simulink model "Vehicle_Model_WIP_V2"  (R2019b)
settings: Solver=FixedStepDiscrete  StartTime=0.0  StopTime=Simulink.t_end  FixedStep=Simulink.dt  RelTol=1e-3
undefined symbols (not defined in the file): BRK, BTRRAD, CHLR, CHRG, DCDC, DiscIntNeverNeededParam, FAN, INV, MTR, PTRAD, PUMP, Settings, TRSM, Vehicle, VHCL, WHL
libraries: simulink x9, EV_cooling x6, EV_VLD x5, EV_ePWT x5
(part 3 of 5)

== system Vehicle_Model_WIP_V2/VCU/Torque Request ==
  note: Regen Braking
  note: Coasting
  note: Regen Braking
  DRV_rThrottle : Inport
  DRV_rBrake : Inport  Port=2
  VLD_vActVhcl_kph : Inport  Port=3
  VCU_LimTrqFr_Nm : Inport  Port=4
  VCU_LimTrqRr_Nm : Inport  Port=5
  HMI_Cruise_kph : Inport  Port=6
  Abs : Abs
  Add : Sum
  BRK_Pct_Brk1 : Lookup_n-D  BreakpointsForDimension1=[0,0.1,0.2,0.5,0.75]  BreakpointsForDimension2=[0,18,72,135]  Table=reshape([0,0,0,0,0,0,0,0,0,0,1,0,0,0,0,1,0,0,0,0],5,4)  ExtrapMethod=Clip  UseLastTableValue=on  RndMeth=Simplest  InputSameDT=on
  Bias : Bias  Bias=-1
  Constant : Constant  Value=MTR.Front.Max_Torque_Nm
  Constant1 : Constant  Value=MTR.Rear.Max_Torque_Nm
  Gain1 : Gain  Gain=MTR.Front.Number_of_Motors
  Gain2 : Gain  Gain=MTR.Rear.Number_of_Motors
  Gain3 : Gain  Gain=MTR.Front.Number_of_Motors
  Gain4 : Gain  Gain=MTR.Rear.Number_of_Motors
  Product3 : Product  Inputs=3
  Product4 : Product  Inputs=3
  Regen : Subsystem  TreatAsAtomicUnit=on
  RegenCoeff : Constant  Value=0
  Saturation : Saturate  UpperLimit=VHCL.TrqDistr  LowerLimit=VHCL.TrqDistr
  Scope : Scope  NumInputPorts=2
  Sum : Sum  Inputs=+++
  Sum1 : Sum  Inputs=+++
  Terminator : Terminator
  TrqDstr : Subsystem  TreatAsAtomicUnit=on
  TrqDstrb MAP : Lookup_n-D  BreakpointsForDimension1=[0,350,500,2360]  BreakpointsForDimension2=[0,150,200,420]  Table=reshape([1,1,0.33,0.33,1,1,0.33,0.33,0.33,0.33,0.33,0.33,0.33,0.33,0.33,0.33],4,4)  InternalRulePriority=Speed  RndMeth=Simplest  InputSameDT=on
  TrqReqFr_Nm : Outport
  TrqReqRr_Nm : Outport  Port=2
  TrqDstrRr : Outport  Port=3
  VCU_rBrk : Outport  Port=4
  wires:
  DRV_rThrottle/1 -> [DRV_rThrottle]
  [DRV_rThrottle] -> TrqDstr/1(DRV_rThrottle)
  DRV_rBrake/1 -> [DRV_rBrake]
  VLD_vActVhcl_kph/1 -> [VLD_vAct]
  HMI_Cruise_kph/1 -> [HMI_Cruise]
  [HMI_Cruise] -> Terminator/1
  [DRV_rThrottle] -> BRK_Pct_Brk1/1
  [VLD_vAct] -> BRK_Pct_Brk1/2
  BRK_Pct_Brk1/1 -> Product3/2, Product4/2
  RegenCoeff/1 -> Product4/1, Product3/3
  [TrqReqFr] -> Sum/1
  [TrqReqRr] -> Sum1/2
  Constant/1 -> Gain3/1
  Constant1/1 -> Gain4/1
  [DRV_rBrake] -> Regen/1(DRV_rBrake)
  Regen/2(BrkTrqReqRr) -> [BrkTrqReqRr]
  Regen/1(BrkTrqReqFr) -> [BrkTrqReqFr]
  [BrkTrqReqFr] -> Sum/2
  Product4/1 -> Sum1/1
  Product3/1 -> Sum/3
  [BrkTrqReqRr] -> Sum1/3
  Regen/3(rBrk) -> VCU_rBrk/1
  [VLD_vAct] -> TrqDstrb MAP/2  "actual speed [km/h]"
  [VLD_vAct] -> Regen/2(VLD_vAct)
  TrqDstr/1(TrqReqFr) -> [TrqReqFr]
  TrqDstr/2(TrqReqRr) -> [TrqReqRr]
  Abs/1 -> TrqDstrRr/1
  Bias/1 -> Abs/1
  TrqDstrb MAP/1 -> Saturation/1  "Torque distribution FRONT [%]"
  [VCU_LimTrqFr_Nm] -> Gain1/1
  [VCU_LimTrqRr_Nm] -> Gain2/1
  [TrqDstrbFr] -> TrqDstr/2(TrqDistrFr)
  [TrqDstrbFr] -> Regen/3(TrqDistrFr)
  Add/1 -> TrqDstrb MAP/1  "Torque request [Nm]"
  Saturation/1 -> Bias/1, [TrqDstrbFr]
  VCU_LimTrqFr_Nm/1 -> [VCU_LimTrqFr_Nm]
  VCU_LimTrqRr_Nm/1 -> [VCU_LimTrqRr_Nm]
  Sum/1 -> Scope/1, TrqReqFr_Nm/1  "TrqReq_FrAxle_Nm"
  Sum1/1 -> Scope/2, TrqReqRr_Nm/1  "TrqReq_RrAxle_Nm"
  Gain1/1 -> Add/1  "Torque request [Nm]"
  Gain2/1 -> Add/2  "Torque request [Nm]"
  Gain3/1 -> Product3/1  "Torque request [Nm]"
  Gain4/1 -> Product4/3  "Torque request [Nm]"

== system Vehicle_Model_WIP_V2/VLD/Front Wheel Radius ==
  Vehicle Actual Speed [m/s] : Inport
  Weight Front [N] : Inport  Port=2
  " Wheel static radius under load" : Subsystem  Commented=on
  Constant{,1,10,15} (4 alike) : Constant
  Constant11 : Constant  Value=VHCL.Front.RollRadius_s1
  Constant12 : Constant  Value=VHCL.Front.RollRadius_s2
  Constant13 : Constant  Value=VHCL.Front.RollRadius_s3
  Constant14 : Constant  Value=VHCL.Front.RollRadius_s4
  Constant16 : Constant  Value=VHCL.Front.RollRadius_c
  Constant2 : Constant  Value=VHCL.Front.RollRadius_q1
  Constant3 : Constant  Value=VHCL.Front.RollRadius_p1
  Constant4 : Constant  Value=VHCL.Front.RollRadius_p2
  Constant5 : Constant  Value=VHCL.Front.RollRadius_p3
  Constant6 : Constant  Value=VHCL.Front.RollRadius_p4
  Constant7 : Constant  Value=VHCL.Front.RollRadius_q2
  Constant8 : Constant  Value=VHCL.Front.RollRadius_q3
  Constant9 : Constant  Value=VHCL.Front.RollRadius_q4
  Divide{1..19} (19 alike) : Product
  Gain : Gain  Gain=0.5
  Goto2 : Goto  Commented=on  GotoTag=LVD_RFrStc_m
  Subtract : Sum  Inputs=4
  Subtract1 : Sum  Inputs=4
  Subtract2 : Sum  Inputs=4
  Subtract3 : Sum  Inputs=3
  LVD_RWhlFr_m : Outport  VectorParamsAs1DForOutWhenUnconnected=off
  wires:
  [LVD_RWhlFr_m] -> LVD_RWhlFr_m/1
  Vehicle Actual Speed [m/s]/1 -> [v_mps]
  " Wheel static radius under load"/1(LVD_RFrStc_m) -> Goto2/1
  Subtract3/1 -> Divide19/2
  [v_mps] -> Divide2/1, Divide2/2
  Divide2/1 -> [v_mps_2]
  Divide4/1 -> [W_N_3]
  Divide5/1 -> Divide4/1, [W_N_2]
  [W_N] -> Divide5/2, Divide4/2, Divide5/1
  Constant3/1 -> Divide1/1
  [W_N_3] -> Divide1/2
  [W_N_2] -> Divide6/2
  Constant4/1 -> Divide6/1
  Constant6/1 -> Divide8/1
  Constant/1 -> Divide8/2
  [W_N] -> Divide7/2
  Constant5/1 -> Divide7/1
  Divide1/1 -> Subtract/1
  Divide6/1 -> Subtract/2
  Divide7/1 -> Subtract/3
  Divide8/1 -> Subtract/4
  Subtract/1 -> Divide9/1
  [v_mps_2] -> Divide9/2
  [v_mps] -> Divide13/2
  Subtract1/1 -> Divide13/1
  Divide12/1 -> Subtract1/4
  Divide11/1 -> Subtract1/3
  Divide10/1 -> Subtract1/2
  Divide3/1 -> Subtract1/1
  Constant8/1 -> Divide11/1
  [W_N] -> Divide11/2
  Constant1/1 -> Divide12/2
  Constant9/1 -> Divide12/1
  Constant7/1 -> Divide10/1
  [W_N_2] -> Divide10/2
  [W_N_3] -> Divide3/2
  Constant2/1 -> Divide3/1
  Constant11/1 -> Divide18/1
  [W_N_3] -> Divide18/2
  [W_N_2] -> Divide14/2
  Constant12/1 -> Divide14/1
  Constant14/1 -> Divide16/1
  Constant10/1 -> Divide16/2
  [W_N] -> Divide15/2
  Constant13/1 -> Divide15/1
  Divide18/1 -> Subtract2/1
  Divide14/1 -> Subtract2/2
  Divide15/1 -> Subtract2/3
  Divide16/1 -> Subtract2/4
  Subtract2/1 -> Divide17/1
  Constant15/1 -> Divide17/2
  Divide9/1 -> Subtract3/1
  Divide13/1 -> Subtract3/2
  Divide17/1 -> Subtract3/3
  Divide19/1 -> [LVD_RWhlFr_m]
  Constant16/1 -> Divide19/1
  Weight Front [N]/1 -> Gain/1
  Gain/1 -> [W_N]

== system Vehicle_Model_WIP_V2/VLD/Inertia ==
  note: Rear
  note: Front
  TRSM_tauFrt : Inport
  TRSM_tauRr : Inport  Port=2
  Add5 : Sum  Inputs=3
  Add6 : Sum  Inputs=3
  Constant1 : Constant  Value=MTR.Front.Number_of_Motors
  Constant11 : Constant  Value=TRSM.Front.Inertia_kgm2
  Constant12 : Constant  Value=TRSM.Rear.Inertia_kgm2
  Constant13 : Constant  Value=MTR.Rear.Inertia_kgm2
  Constant14 : Constant  Value=WHL.Rear.Inertia_kgm2
  Constant2 : Constant  Value=MTR.Rear.Number_of_Motors
  Constant3 : Constant  Value=MTR.Front.Number_of_Motors
  Constant4 : Constant  Value=MTR.Rear.Number_of_Motors
  Constant8 : Constant  Value=MTR.Front.Inertia_kgm2
  Constant9 : Constant  Value=WHL.Front.Inertia_kgm2
  Divide{1,5,8,10} (4 alike) : Product
  Divide{2..3,7,11} (4 alike) : Product  Inputs=3
  Gain2 : Gain  Gain=2
  Gain3 : Gain  Gain=2
  VLD_FrtInrt_kgm2 : Outport  VectorParamsAs1DForOutWhenUnconnected=off
  VLD_RrInrt_kgm2 : Outport  Port=2  VectorParamsAs1DForOutWhenUnconnected=off
  wires:
  TRSM_tauFrt/1 -> [TRSM_tauFrt]
  TRSM_tauRr/1 -> [TRSM_tauRr]
  Divide5/1 -> Divide7/1
  Constant8/1 -> Divide7/2
  [TRSM_tauFrt] -> Divide5/2, Divide5/1
  Divide1/1 -> Divide2/1
  [TRSM_tauFrt] -> Divide1/1, Divide1/2
  Constant11/1 -> Divide2/2
  Constant9/1 -> Gain2/1
  Divide2/1 -> Add5/2
  Gain2/1 -> Add5/3
  Divide7/1 -> Add5/1
  Constant14/1 -> Gain3/1
  Divide11/1 -> Add6/1
  Constant13/1 -> Divide11/2
  [TRSM_tauRr] -> Divide8/1, Divide8/2
  Gain3/1 -> Add6/3
  Divide10/1 -> Divide11/1
  [TRSM_tauRr] -> Divide10/2, Divide10/1
  Add5/1 -> [VLD_FrtInrt_kgm2]
  Add6/1 -> [VLD_RrInrt_kgm2]
  [VLD_RrInrt_kgm2] -> VLD_RrInrt_kgm2/1
  [VLD_FrtInrt_kgm2] -> VLD_FrtInrt_kgm2/1
  Constant1/1 -> Divide7/3
  Constant2/1 -> Divide11/3
  Constant3/1 -> Divide2/3
  Divide3/1 -> Add6/2
  Constant12/1 -> Divide3/2
  Divide8/1 -> Divide3/1
  Constant4/1 -> Divide3/3

== system Vehicle_Model_WIP_V2/VLD/Rear Wheel Radius ==
  Vehicle Actual Speed [m/s] : Inport
  Weight Rear [N] : Inport  Port=2
  " Wheel static radius under load" : Subsystem  Commented=on
  Constant{,1,10,15} (4 alike) : Constant
  Constant11 : Constant  Value=VHCL.Rear.RollRadius_s1
  Constant12 : Constant  Value=VHCL.Rear.RollRadius_s2
  Constant13 : Constant  Value=VHCL.Rear.RollRadius_s3
  Constant14 : Constant  Value=VHCL.Rear.RollRadius_s4
  Constant16 : Constant  Value=VHCL.Rear.RollRadius_c
  Constant2 : Constant  Value=VHCL.Rear.RollRadius_q1
  Constant3 : Constant  Value=VHCL.Rear.RollRadius_p1
  Constant4 : Constant  Value=VHCL.Rear.RollRadius_p2
  Constant5 : Constant  Value=VHCL.Rear.RollRadius_p3
  Constant6 : Constant  Value=VHCL.Rear.RollRadius_p4
  Constant7 : Constant  Value=VHCL.Rear.RollRadius_q2
  Constant8 : Constant  Value=VHCL.Rear.RollRadius_q3
  Constant9 : Constant  Value=VHCL.Rear.RollRadius_q4
  Divide{1..19} (19 alike) : Product
  Gain : Gain  Gain=0.5
  Goto2 : Goto  Commented=on  GotoTag=LVD_RFrStc_m
  Subtract : Sum  Inputs=4
  Subtract1 : Sum  Inputs=4
  Subtract2 : Sum  Inputs=4
  Subtract3 : Sum  Inputs=3
  LVD_RWhlRr_m : Outport  VectorParamsAs1DForOutWhenUnconnected=off
  wires:
  [LVD_RWhlFr_m] -> LVD_RWhlRr_m/1
  Vehicle Actual Speed [m/s]/1 -> [v_mps]
  " Wheel static radius under load"/1(LVD_RFrStc_m) -> Goto2/1
  [v_mps] -> Divide2/1, Divide2/2
  Divide2/1 -> [v_mps_2]
  Divide4/1 -> [W_N_3]
  Divide5/1 -> Divide4/1, [W_N_2]
  [W_N] -> Divide5/2, Divide4/2, Divide5/1
  Constant3/1 -> Divide1/1
  [W_N_3] -> Divide1/2
  [W_N_2] -> Divide6/2
  Constant4/1 -> Divide6/1
  Constant6/1 -> Divide8/1
  Constant/1 -> Divide8/2
  [W_N] -> Divide7/2
  Constant5/1 -> Divide7/1
  Divide1/1 -> Subtract/1
  Divide6/1 -> Subtract/2
  Divide7/1 -> Subtract/3
  Divide8/1 -> Subtract/4
  Subtract/1 -> Divide9/1
  [v_mps_2] -> Divide9/2
  [v_mps] -> Divide13/2
  Subtract1/1 -> Divide13/1
  Divide12/1 -> Subtract1/4
  Divide11/1 -> Subtract1/3
  Divide10/1 -> Subtract1/2
  Divide3/1 -> Subtract1/1
  Constant8/1 -> Divide11/1
  [W_N] -> Divide11/2
  Constant1/1 -> Divide12/2
  Constant9/1 -> Divide12/1
  Constant7/1 -> Divide10/1
  [W_N_2] -> Divide10/2
  [W_N_3] -> Divide3/2
  Constant2/1 -> Divide3/1
  Constant11/1 -> Divide18/1
  [W_N_3] -> Divide18/2
  [W_N_2] -> Divide14/2
  Constant12/1 -> Divide14/1
  Constant14/1 -> Divide16/1
  Constant10/1 -> Divide16/2
  [W_N] -> Divide15/2
  Constant13/1 -> Divide15/1
  Divide18/1 -> Subtract2/1
  Divide14/1 -> Subtract2/2
  Divide15/1 -> Subtract2/3
  Divide16/1 -> Subtract2/4
  Subtract2/1 -> Divide17/1
  Constant15/1 -> Divide17/2
  Divide9/1 -> Subtract3/1
  Divide13/1 -> Subtract3/2
  Divide17/1 -> Subtract3/3
  Divide19/1 -> [LVD_RWhlFr_m]
  Constant16/1 -> Divide19/1
  Subtract3/1 -> Divide19/2
  Weight Rear [N]/1 -> Gain/1
  Gain/1 -> [W_N]

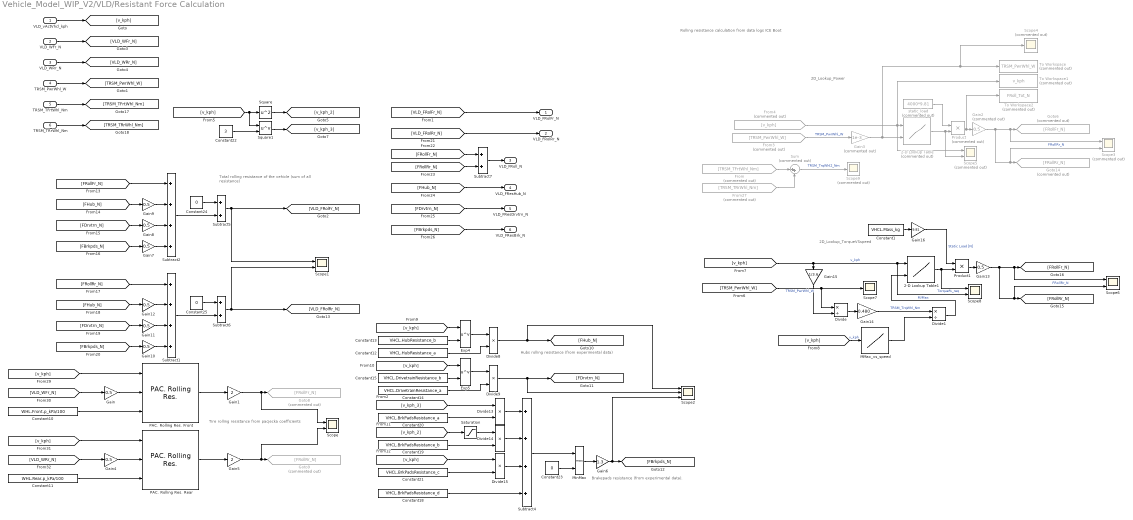
== system Vehicle_Model_WIP_V2/VLD/Resistant Force Calculation ==
  note: Rolling resistance calculation from data logs ICE Boot
  note: 2D_Lookup_Power
  note: Hubs rolling resistance (from experimental data)
  note: Brakepads resistance (from experimental data).
  note: Tire rolling resistance from pacjecka coefficients
  note: Total rolling resistance of the vehicle (sum of all resistance)
  note: 2D_Lookup_TorqueVSspeed
  VLD_vActVhcl_kph : Inport
  VLD_WFr_N : Inport  Port=2
  VLD_WRr_N : Inport  Port=3
  TRSM_PwrWhl_W : Inport  Port=4
  TRSM_TFrtWhl_Nm : Inport  Port=5
  TRSM_TRrWhl_Nm : Inport  Port=6
  2-D Lookup Table : Lookup_n-D  Commented=on  BreakpointsForDimension1=[0,1,18,54,72,162]  BreakpointsForDimension2=[0,250]  Table=reshape([0,0.23,0.23,0.18,0.15,0.15,0.68,0.68,0.68,0.3,0.3,0.3],6,2)  ExtrapMethod=Clip  InternalRulePriority=Speed  RndMeth=Simplest  InputSameDT=on
  2-D Lookup Table1 : Lookup_n-D  BreakpointsForDimension1=[0,1,18,54,72,162]  BreakpointsForDimension2=[0,1.4,2]  Table=reshape([0,0.23,0.23,0.18,0.15,0.15,0.68,0.68,0.68,0.3,0.3,0.3,0.75,0.75,0.75,0.35,0.35,0.35],6,3)  ExtrapMethod=Clip  InternalRulePriority=Speed  RndMeth=Simplest  InputSameDT=on
  Constant1 : Constant  Value=VHCL.Mass_kg  VectorParams1D=off
  Constant10 : Constant  Value=WHL.Front.p_kPa/100
  Constant11 : Constant  Value=WHL.Rear.p_kPa/100
  Constant12 : Constant  Value=VHCL.HubResistance_a
  Constant13 : Constant  Value=VHCL.HubResistance_b
  Constant14 : Constant  Value=VHCL.DrivetrainResistance_a
  Constant15 : Constant  Value=VHCL.DrivetrainResistance_b
  Constant18 : Constant  Value=VHCL.BrkPadsResistance_d
  Constant19 : Constant  Value=VHCL.BrkPadsResistance_b
  Constant20 : Constant  Value=VHCL.BrkPadsResistance_a
  Constant21 : Constant  Value=VHCL.BrkPadsResistance_c
  Constant22 : Constant  Value=3
  Constant23 : Constant  Value=0
  Constant24 : Constant  Value=0
  Constant25 : Constant  Value=0
  Divide : Product  Inputs=*/
  Divide1 : Product  Inputs=*/
  Divide{8..9,13..15} (5 alike) : Product
  Exp4 : Math  Operator=pow  SignedPower=off  SaturateOnIntegerOverflow=on
  Exp5 : Math  Operator=pow  SignedPower=off  SaturateOnIntegerOverflow=on
  From : From  Commented=on  GotoTag=TRSM_TFrtWhl_Nm
  From27 : From  Commented=on  GotoTag=TRSM_TRrWhl_Nm
  From3 : From  Commented=on  GotoTag=TRSM_PwrWhl_W
  From4 : From  Commented=on  GotoTag=v_kph
  Gain{,4,7..13} (9 alike) : Gain  Gain=0.5
  Gain1 : Gain  Gain=2
  Gain14 : Gain  Gain=0.480
  Gain15 : Gain  Gain=1/3.6
  Gain16 : Gain  Gain=9.81
  Gain2 : Gain  Commented=on  Gain=0.5
  Gain3 : Gain  Commented=on  Gain=1e-3
  Gain5 : Gain  Gain=2
  Gain6 : Gain  Gain=1.3
  Goto14 : Goto  Commented=on  GotoTag=FRollRr_N
  Goto6 : Goto  Commented=on  GotoTag=FRollFr_N
  Goto8 : Goto  Commented=on  GotoTag=FRollFr_N
  Goto9 : Goto  Commented=on  GotoTag=FRollRr_N
  MMax_vs_speed : Lookup_n-D  NumberOfTableDimensions=1  BreakpointsForDimension1=[0 5 10 15 20 25 30 35 40 45]*3.6  Table=[17000 17000 9500 7500 5750 4750 4000 3250 2800 2500]  ExtrapMethod=Clip  InternalRulePriority=Speed  RndMeth=Simplest  InputSameDT=on
  MinMax : MinMax  Function=max  Inputs=2
  PAC. Rolling Res. Front : EV_VLD/PAC. Rolling Res.  Vref_kmph=VHCL.RollResistance_V0  Fzref_N=VHCL.RollResistance_Fz0  pref_bar=VHCL.RollResistance_p0  SF=VHCL.Front.CRRgain  qsy1=VHCL.RollResistance_qsy1  qsy2=VHCL.RollResistance_qsy2  qsy3=VHCL.RollResistance_qsy3  qsy4=VHCL.RollResistance_qsy4  qsy5=VHCL.RollResistance_qsy5  qsy6=VHCL.RollResistance_qsy6  qsy7=VHCL.RollResistance_qsy7  qsy8=VHCL.RollResistance_qsy8
      settings: SourceProductName=EV_lib
  PAC. Rolling Res. Rear : EV_VLD/PAC. Rolling Res.  Vref_kmph=VHCL.RollResistance_V0  Fzref_N=VHCL.RollResistance_Fz0  pref_bar=VHCL.RollResistance_p0  SF=VHCL.Rear.CRRgain  qsy1=VHCL.RollResistance_qsy1  qsy2=VHCL.RollResistance_qsy2  qsy3=VHCL.RollResistance_qsy3  qsy4=VHCL.RollResistance_qsy4  qsy5=VHCL.RollResistance_qsy5  qsy6=VHCL.RollResistance_qsy6  qsy7=VHCL.RollResistance_qsy7  qsy8=VHCL.RollResistance_qsy8
      settings: SourceProductName=EV_lib
  Product : Product  Commented=on
  Product1 : Product
  Saturation : Saturate  UpperLimit=150*150  LowerLimit=0
  Scope{,1,6,8} (4 alike) : Scope  NumInputPorts=2
  Scope2 : Scope  NumInputPorts=3
  Scope3 : Scope  Commented=on  NumInputPorts=2
  Scope4 : Scope  Commented=on
  Scope5 : Scope  Commented=on  NumInputPorts=2
  Scope7 : Scope
  Scope9 : Scope  Commented=on
  Square : Math  Operator=square  SignedPower=off  SaturateOnIntegerOverflow=on
  Square1 : Math  Operator=pow  SignedPower=off  SaturateOnIntegerOverflow=on
  Subtract1 : Sum  Inputs=++++
  Subtract2 : Sum  Inputs=++++
  Subtract4 : Sum  Inputs=++++
  Subtract5 : Sum
  Subtract6 : Sum
  Subtract7 : Sum
  Sum : Sum  Commented=on  Inputs=|++
  To Workspace : ToWorkspace  Commented=on  VariableName=TRSM_PwrWhl_W  SaveFormat=Timeseries  SampleTime=-1
  To Workspace1 : ToWorkspace  Commented=on  VariableName=v_kph  SaveFormat=Timeseries  SampleTime=-1
  To Workspace2 : ToWorkspace  Commented=on  VariableName=FRoll_Tot_N  SaveFormat=Timeseries  SampleTime=-1
  static_load : Constant  Commented=on  Value=4000*9.81
  VLD_FRolFr_N : Outport  VectorParamsAs1DForOutWhenUnconnected=off
  VLD_FRolRr_N : Outport  Port=2  VectorParamsAs1DForOutWhenUnconnected=off
  VLD_FRoll_N : Outport  Port=3  VectorParamsAs1DForOutWhenUnconnected=off
  VLD_FResHub_N : Outport  Port=4  VectorParamsAs1DForOutWhenUnconnected=off
  VLD_FResDrvtrn_N : Outport  Port=5  VectorParamsAs1DForOutWhenUnconnected=off
  VLD_FResBrk_N : Outport  Port=6  VectorParamsAs1DForOutWhenUnconnected=off
  wires:
  VLD_vActVhcl_kph/1 -> [v_kph]
  [VLD_FRolFr_N] -> VLD_FRolFr_N/1
  [v_kph] -> Square1/1, Square/1
  Square/1 -> [v_kph_2]
  VLD_WFr_N/1 -> [VLD_WFr_N]
  VLD_WRr_N/1 -> [VLD_WRr_N]
  Constant12/1 -> Divide8/2
  [v_kph] -> Exp4/1
  Constant13/1 -> Exp4/2
  Exp4/1 -> Divide8/1
  Exp5/1 -> Divide9/1
  Constant15/1 -> Exp5/2
  [v_kph] -> Exp5/1
  Constant14/1 -> Divide9/2
  Constant18/1 -> Subtract4/4
  Divide13/1 -> Subtract4/1
  Divide14/1 -> Subtract4/2
  [v_kph_2] -> Saturation/1
  Constant19/1 -> Divide14/2
  Constant20/1 -> Divide13/2
  [v_kph_3] -> Divide13/1
  Constant21/1 -> Divide15/2
  [v_kph] -> Divide15/1
  Divide15/1 -> Subtract4/3
  Square1/1 -> [v_kph_3]
  Constant22/1 -> Square1/2
  MinMax/1 -> Gain6/1
  Subtract4/1 -> MinMax/1
  Constant23/1 -> MinMax/2
  Subtract5/1 -> [VLD_FRolFr_N], Scope1/1
  Subtract2/1 -> Subtract5/2
  Constant24/1 -> Subtract5/1
  Divide8/1 -> [FHub_N], Scope2/1
  Divide9/1 -> [FDrvtrn_N], Scope2/2
  Gain6/1 -> [FBrkpds_N], Scope2/3
  [FRollFr_N] -> Subtract2/1
  [FHub_N] -> Gain9/1
  [FDrvtrn_N] -> Gain8/1
  [FBrkpds_N] -> Gain7/1
  Gain7/1 -> Subtract2/4
  Gain8/1 -> Subtract2/3
  Gain9/1 -> Subtract2/2
  Gain12/1 -> Subtract1/2
  Gain11/1 -> Subtract1/3
  Gain10/1 -> Subtract1/4
  [FBrkpds_N] -> Gain10/1
  [FDrvtrn_N] -> Gain11/1
  [FHub_N] -> Gain12/1
  [FRollRr_N] -> Subtract1/1
  Constant25/1 -> Subtract6/1
  Subtract1/1 -> Subtract6/2
  Subtract6/1 -> [VLD_FRolRr_N], Scope1/2
  [VLD_FRolRr_N] -> VLD_FRolRr_N/1
  [FRollRr_N] -> Subtract7/2
  [FRollFr_N] -> Subtract7/1
  Subtract7/1 -> VLD_FRoll_N/1
  Saturation/1 -> Divide14/1
  [FHub_N] -> VLD_FResHub_N/1
  [FDrvtrn_N] -> VLD_FResDrvtrn_N/1
  [FBrkpds_N] -> VLD_FResBrk_N/1
  [v_kph] -> PAC. Rolling Res. Front/1
  [VLD_WFr_N] -> Gain/1
  Gain/1 -> PAC. Rolling Res. Front/2
  Constant10/1 -> PAC. Rolling Res. Front/3
  PAC. Rolling Res. Front/1 -> Gain1/1
  PAC. Rolling Res. Rear/1 -> Gain5/1
  Constant11/1 -> PAC. Rolling Res. Rear/3
  Gain4/1 -> PAC. Rolling Res. Rear/2
  [VLD_WRr_N] -> Gain4/1
  [v_kph] -> PAC. Rolling Res. Rear/1
  Gain1/1 -> Scope/1, Goto8/1
  Gain5/1 -> Scope/2, Goto9/1
  TRSM_PwrWhl_W/1 -> [TRSM_PwrWhl_W]
  Product/1 -> To Workspace2/1, Gain2/1
  Gain2/1 -> Scope3/1, Goto6/1, Scope3/2, Goto14/1  "FRollRr_N"
  From3/1 -> Gain3/1  "TRSM_PwrWhl_W"
  From4/1 -> Scope5/1, 2-D Lookup Table/1, To Workspace1/1
  2-D Lookup Table/1 -> Scope5/2, Product/2
  static_load/1 -> Product/1
  Gain3/1 -> 2-D Lookup Table/2, To Workspace/1, Scope4/1
  Gain16/1 -> Product1/1  "Static Load [N]"
  2-D Lookup Table1/1 -> Product1/2, Scope8/1  "Torque%_req"
  [v_kph] -> 2-D Lookup Table1/1, Scope8/2, Gain15/1  "v_kph"
  [TRSM_PwrWhl_W] -> Scope7/1, Divide/1  "TRSM_PwrWhl_W"
  Gain13/1 -> [FRollRr_N], Scope6/2, [FRollFr_N], Scope6/1  "FRollRr_N"
  Product1/1 -> Gain13/1
  Divide/1 -> Gain14/1
  Gain14/1 -> Divide1/1  "TRSM_TrqWhl_Nm"
  [v_kph] -> MMax_vs_speed/1  "v_kph"
  MMax_vs_speed/1 -> Divide1/2
  Divide1/1 -> 2-D Lookup Table1/2  "M/Max"
  TRSM_TFrtWhl_Nm/1 -> [TRSM_TFrtWhl_Nm]
  TRSM_TRrWhl_Nm/1 -> [TRSM_TRrWhl_Nm]
  From/1 -> Sum/1
  From27/1 -> Sum/2
  Sum/1 -> Scope9/1  "TRSM_TrqWhl2_Nm"
  Gain15/1 -> Divide/2
  Constant1/1 -> Gain16/1

== system Vehicle_Model_WIP_V2/VLD/old ==
  In1 : Inport
  In2 : Inport  Port=2
  In3 : Inport  Port=3
  In4 : Inport  Port=4
  In5 : Inport  Port=5
  In6 : Inport  Port=6
  In7 : Inport  Port=7
  In8 : Inport  Port=8
  In9 : Inport  Port=9
  In10 : Inport  Port=10
  In11 : Inport  Port=11
  In12 : Inport  Port=12
  In13 : Inport  Port=13
  In14 : Inport  Port=14
  In15 : Inport  Port=15
  In16 : Inport  Port=16
  In17 : Inport  Port=17
  In18 : Inport  Port=18
  In19 : Inport  Port=19
  In20 : Inport  Port=20
  In21 : Inport  Port=21
  In22 : Inport  Port=22
  In23 : Inport  Port=23
  In24 : Inport  Port=24
  In25 : Inport  Port=25
  In26 : Inport  Port=26
  OLD VLD : Subsystem  Commented=on
  Slope Force Calculation1 : Subsystem  Commented=on
  Vehicle force and power calculation : Subsystem  Commented=on
  Weigth Distribution Front1 : Subsystem  Commented=on
  Weigth Distribution Rear1 : Subsystem  Commented=on
  Out1 : Outport
  Out2 : Outport  Port=2
  Out3 : Outport  Port=3
  Out4 : Outport  Port=4
  Out5 : Outport  Port=5
  Out6 : Outport  Port=6
  Out7 : Outport  Port=7
  Out8 : Outport  Port=8
  Out9 : Outport  Port=9
  Out10 : Outport  Port=10
  Out11 : Outport  Port=11
  Out12 : Outport  Port=12
  Out13 : Outport  Port=13
  Out14 : Outport  Port=14
  Out15 : Outport  Port=15
  Out16 : Outport  Port=16
  Out17 : Outport  Port=17
  Out18 : Outport  Port=18
  Out19 : Outport  Port=19
  Out20 : Outport  Port=20
  Out21 : Outport  Port=21
  Out22 : Outport  Port=22
  Out23 : Outport  Port=23
  Out24 : Outport  Port=24
  Out25 : Outport  Port=25
  Out26 : Outport  Port=26
  Out27 : Outport  Port=27
  wires:
  Vehicle force and power calculation/3(VLD_FTot_N) -> Out17/1
  In11/1 -> Vehicle force and power calculation/1(LVD_RWhlFr_m)
  OLD VLD/2(v_mps) -> Out6/1
  OLD VLD/7(vWRr_mps) -> Out11/1
  Weigth Distribution Front1/1(VLD_WDisrtFr_N) -> Out3/1
  In20/1 -> Vehicle force and power calculation/10(VLD_FRes_N)
  Slope Force Calculation1/2(VLD_Wtot_N) -> Out2/1
  Vehicle force and power calculation/2(VLD_FRst_N) -> Out16/1
  In23/1 -> Vehicle force and power calculation/13(VLD_FRoll_N)
  OLD VLD/1(l_km) -> Out5/1
  In9/1 -> Weigth Distribution Front1/4(Vehicle Actual Speed [m/s])
  Vehicle force and power calculation/7(VLD_PTot_W) -> Out21/1
  OLD VLD/3(a_mps2) -> Out7/1
  Slope Force Calculation1/1(VLD_FSlp_N) -> Out1/1
  OLD VLD/9(slipRr) -> Out13/1
  In2/1 -> Slope Force Calculation1/2(INPT_sReq_Pct)
  Vehicle force and power calculation/4(VLD_FInrt_N) -> Out18/1
  In8/1 -> Weigth Distribution Rear1/3("Vehicle Actual Acc [m/s2] ")
  In13/1 -> Vehicle force and power calculation/3(TRSM_TFrtWhl_Nm)
  OLD VLD/6(nWRr_RPM) -> Out10/1
  OLD VLD/8(slipFr) -> Out12/1
  Vehicle force and power calculation/8(VLD_PInrt_W) -> Out22/1
  OLD VLD/4(nWFr_RPM) -> Out8/1
  Vehicle force and power calculation/1(VLD_FWhl_N) -> Out15/1
  OLD VLD/10(slipLoss_W) -> Out14/1
  Vehicle force and power calculation/11(VLD_PResDrvtrn_W) -> Out25/1
  In14/1 -> Vehicle force and power calculation/4(TRSM_TRrWhl_Nm)
  In19/1 -> Vehicle force and power calculation/9(VLD_FRolRr_N)
  OLD VLD/5(vWFr_mps) -> Out9/1
  In1/1 -> Slope Force Calculation1/1(VLD_mReal_kg)
  Vehicle force and power calculation/12(VLD_PResBrk_W) -> Out26/1
  In17/1 -> Vehicle force and power calculation/7(VLD_FSlp_N)
  In12/1 -> Vehicle force and power calculation/2(LVD_RWhlRr_m)
  In15/1 -> Vehicle force and power calculation/5(BRK_TFrt_Nm)
  In16/1 -> Vehicle force and power calculation/6(BRK_TRr_Nm)
  In26/1 -> Vehicle force and power calculation/16(VLD_FResBrk_N)
  In22/1 -> Vehicle force and power calculation/12(VLD_mEquiv_kg)
  In24/1 -> Vehicle force and power calculation/14(VLD_FResHub_N)
  Vehicle force and power calculation/13(VLD_PDrag_W) -> Out27/1
  In21/1 -> Vehicle force and power calculation/11(VLD_vActVhcl_kph)
  In25/1 -> Vehicle force and power calculation/15(VLD_FResDrvtrn_N)
  In18/1 -> Vehicle force and power calculation/8(VLD_FRolFr_N)
  Vehicle force and power calculation/5(VLD_PWhl_W) -> Out19/1
  In4/1 -> Weigth Distribution Rear1/1(Mass real [kg])
  In7/1 -> Weigth Distribution Front1/3("Vehicle Actual Acc [m/s2] ")
  Vehicle force and power calculation/6(VLD_PRst_W) -> Out20/1
  In5/1 -> Weigth Distribution Front1/2(WTot_N)
  Vehicle force and power calculation/10(VLD_PRoll_W) -> Out24/1
  Vehicle force and power calculation/9(VLD_PWhlMtr_W) -> Out23/1
  In3/1 -> Weigth Distribution Front1/1(Mass real [kg])
  Weigth Distribution Rear1/1(VLD_WDisrtRr_N) -> Out4/1
  In10/1 -> Weigth Distribution Rear1/4(Vehicle Actual Speed [m/s])
  In6/1 -> Weigth Distribution Rear1/2(WTot_N)

== system Vehicle_Model_WIP_V2/old cooling/Battery Cooling system ==
  note: Low Temperature Radiator
  note: Chiller
  note: Battery cooling system:
      | Chiller and radiator models.
  INIT : Inport
  BTR : Inport  Port=2
  VCU : Inport  Port=3
  FAN : Inport  Port=4
  Battery Pack Chiller : Subsystem
  Bus Creator : BusCreator  Inputs=7
  Bus Selector : BusSelector  OutputSignals=BTR_TWtrOut_degC
  Bus Selector1 : BusSelector  OutputSignals=INIT_TSys_degC,INIT_TEnv_degC
  Bus Selector2 : BusSelector  OutputSignals=RAD_dmAir_kgps,RAD_VAirTot_mps
  Bus Selector3 : BusSelector  OutputSignals=VCU_dVBtr_lpm,VCU_bRadLowEnbl,VCU_bChlrEnbl
  Delay2 : Delay  DelayLength=1  InitialConditionSource=Input port
      settings: InputPortMap=u0,p4
  Low Temperature Radiator : Subsystem
  Pump Inertia : Subsystem
  Pump Input Power [W] : Lookup_n-D  NumberOfTableDimensions=1  BreakpointsForDimension1=PUMP.BCS.dV_bp  BreakpointsForDimension2=INV.Front.bp_Torque_Nm_Mtr  BreakpointsForDimension3=MTR.Front.bp_time  Table=PUMP.BCS.Power  ExtrapMethod=Clip  UseLastTableValue=on  RndMeth=Simplest  InputSameDT=on
  BCS : Outport  VectorParamsAs1DForOutWhenUnconnected=off
  wires:
  Bus Creator/1 -> BCS/1
  INIT/1 -> Bus Selector1/1
  Bus Selector1/1 -> [INIT_TSys_degC]  "<INIT_TSys_degC>"
  Bus Selector/1 -> [BTR_TWtrOut_degC]  "<BTR_TWtrOut_degC>"
  BTR/1 -> Bus Selector/1
  [BCS_PHeatRejRad_W] -> Bus Creator/2  "BCS_PHeatRejRad_W"
  [BCS_PHeatRejChlr_W] -> Bus Creator/3  "BCS_PHeatRejChlr_W"
  [BCS_PElec_W] -> Bus Creator/4  "BCS_PElec_W"
  [INIT_TEnv_degC] -> Low Temperature Radiator/3(INPT_TEnv_degC)
  [VCU_bRadLowEnbl] -> Low Temperature Radiator/4(reset)
  [INIT_TSys_degC] -> Battery Pack Chiller/3(INIT_TSys_degC)
  Battery Pack Chiller/3(CHLR_PElec_W) -> [CHLR_PElec_W]
  Battery Pack Chiller/2(CHLR_TWtrOut_degC) -> [CHLR_TWtrOut_degC]
  [BCS_dV_lpm] -> Battery Pack Chiller/2(INIT_dVBtr_lpm)
  Battery Pack Chiller/1(CHLR_PHeatRej_W) -> [CHLR_PHeatRej_W]
  [BCS_dV_lpm] -> Low Temperature Radiator/2(INIT_dVBtr_lpm)
  Low Temperature Radiator/1(RAD_TWtrOut_degC) -> [RAD_TWtrOut_degC]
  [BTR_TWtrOut_degC] -> Low Temperature Radiator/1(BTR_TWtrOut_degC)
  [CHLR_TWtrIn_degC] -> Battery Pack Chiller/1(RAD_TWtrOut_degC)
  Low Temperature Radiator/2(RAD_PHeatRej_W) -> [RAD_PHeatRej_W]
  [CHLR_PHeatRej_W] -> [BCS_PHeatRejChlr_W]
  [CHLR_TWtrOut_degC] -> [BCS_TWtrOut_degC]
  [RAD_PHeatRej_W] -> [BCS_PHeatRejRad_W]
  [CHLR_PElec_W] -> [BCS_PElec_W]
  [RAD_TWtrOut_degC] -> Delay2/1
  Bus Selector1/2 -> [INIT_TEnv_degC]  "<INIT_TEnv_degC>"
  VCU/1 -> Bus Selector3/1
  Bus Selector3/1 -> [VCU_dVBtr_lpm]  "<VCU_dVBtr_lpm>"
  Bus Selector3/2 -> [VCU_bRadLowEnbl]  "<VCU_bRadLowEnbl>"
  Bus Selector3/3 -> [VCU_bChlrEnbl]  "<VCU_bChlrEnbl>"
  Delay2/1 -> [CHLR_TWtrIn_degC]
  [INIT_TSys_degC] -> Delay2/2
  [BCS_dV_lpm] -> Bus Creator/5  "BCS_dV_lpm"
  [VCU_bChlrEnbl] -> Battery Pack Chiller/4(VCU_bChlrEnbl)
  [BCS_TWtrOut_degC] -> Bus Creator/1  "BCS_TWtrOut_degC"
  Low Temperature Radiator/3(RAD_TAirOut_degC) -> [RAD_TAirOut_degC]
  [RAD_TAirOut_degC] -> Bus Creator/6  "BCS_TAirOut_degC"
  [RAD_dmAir_kgps] -> Low Temperature Radiator/5(RAD_dmAir_kgps)
  FAN/1 -> Bus Selector2/1
  Bus Selector2/1 -> [RAD_dmAir_kgps]  "<RAD_dmAir_kgps>"
  Bus Selector2/2 -> [RAD_VAirTot_mps]  "<RAD_VAirTot_mps>"
  [RAD_VAirTot_mps] -> Low Temperature Radiator/6(RAD_vAir_mps)
  [VCU_dVBtr_lpm] -> Pump Input Power [W]/1, Pump Inertia/1(VCU_dVBtr_lpm)
  Pump Input Power [W]/1 -> [BCS_PumpPwr_W]
  [BCS_PumpPwr_W] -> Bus Creator/7  "BCS_PumpPwr_W"
  Pump Inertia/1(BCS_dV_lpm) -> [BCS_dV_lpm]

== system Vehicle_Model_WIP_V2/old cooling/Fan and air for Radiators ==
  note: Air Flow and Fan
  note: Fan and air speed input for radiators.
  INIT : Inport
  VLD : Inport  Port=2
  VCU : Inport  Port=3
  Air Flow and Fan Model : Subsystem
  Bus Creator : BusCreator  Inputs=3
  Bus Selector1 : BusSelector  OutputSignals=INIT_TEnv_degC
  Bus Selector2 : BusSelector  OutputSignals=VLD_vActVhcl_kph
  Bus Selector3 : BusSelector  OutputSignals=VCU_bFanEnblPTCS,VCU_rFanFlow
  FAN : Outport
  wires:
  [INIT_TEnv_degC] -> Air Flow and Fan Model/2(INPT_TEnv_degC)
  [VLD_vActVhcl_kph] -> Air Flow and Fan Model/1(VLD_vActVhcl_kph)
  [VCU_bFanEnblPTCS] -> Air Flow and Fan Model/3(VCU_bFanEnblPTCS)
  Air Flow and Fan Model/1(RAD_dmAir_kgps) -> [RAD_dmAir_kgps]
  VLD/1 -> Bus Selector2/1
  Bus Selector2/1 -> [VLD_vActVhcl_kph]  "<VLD_vActVhcl_kph>"
  VCU/1 -> Bus Selector3/1
  INIT/1 -> Bus Selector1/1
  Bus Selector1/1 -> [INIT_TEnv_degC]  "<INIT_TEnv_degC>"
  Bus Selector3/1 -> [VCU_bFanEnblPTCS]  "<VCU_bFanEnblPTCS>"
  Bus Creator/1 -> FAN/1
  [RAD_dmAir_kgps] -> Bus Creator/1  "RAD_dmAir_kgps"
  Air Flow and Fan Model/2(RAD_VAirTot_mps) -> [RAD_VAirTot_mps]
  [RAD_VAirTot_mps] -> Bus Creator/2  "RAD_VAirTot_mps"
  [VCU_rFanFlow] -> Air Flow and Fan Model/4(VCU_rFanFlow)
  Bus Selector3/2 -> [VCU_rFanFlow]  "<VCU_rFanFlow>"
  Air Flow and Fan Model/3(Fan_PwrReq_W) -> [Fan_PwrReq_W]
  [Fan_PwrReq_W] -> Bus Creator/3  "Fan_PwrReq_W"

== system Vehicle_Model_WIP_V2/old cooling/PowerTrain Cooling system ==
  note: High Temperature Radiator
  note: Power train cooling system:
      | Radiator model.
  FAN : Inport
  INIT : Inport  Port=2
  MTR : Inport  Port=3
  VCU : Inport  Port=4
  BCS : Inport  Port=5
  Add : Sum
  Bus Creator : BusCreator  Inputs=7
  Bus Selector1 : BusSelector  OutputSignals=INIT_TSys_degC
  Bus Selector2 : BusSelector  OutputSignals=RAD_dmAir_kgps,RAD_VAirTot_mps
  Bus Selector3 : BusSelector  OutputSignals=MTR_TWtrOutRr_degC
  Bus Selector4 : BusSelector  OutputSignals=VCU_rFlowMtrFr,VCU_rFlowMtrRr,VCU_dVPwrT_lpm
  Bus Selector5 : BusSelector  OutputSignals=BCS_TAirOut_degC
  Delay : Delay  DelayLength=1  InitialConditionSource=Input port
      settings: InputPortMap=u0,p4
  Divide5 : Product  Inputs=**
  Divide6 : Product  Inputs=**
  Low Temperature Radiator : Subsystem
  Pump Inertia : Subsystem
  Pump Input Power [W] : Lookup_n-D  NumberOfTableDimensions=1  BreakpointsForDimension1=PUMP.PTCS.dV_bp  BreakpointsForDimension2=INV.Front.bp_Torque_Nm_Mtr  BreakpointsForDimension3=MTR.Front.bp_time  Table=PUMP.PTCS.Power  ExtrapMethod=Clip  UseLastTableValue=on  RndMeth=Simplest  InputSameDT=on
  PTCS : Outport  VectorParamsAs1DForOutWhenUnconnected=off
  wires:
  Bus Creator/1 -> PTCS/1
  INIT/1 -> Bus Selector1/1
  [RADBCS_TAirOut_degC] -> Low Temperature Radiator/4(RADBCS_TAirOut_degC)
  [RAD_dVPwr_lpm] -> Low Temperature Radiator/2(INIT_dVPwrT_lpm)
  [RAD_dmAir_kgps] -> Low Temperature Radiator/3(RAD_dmAir_kgps)
  MTR/1 -> Bus Selector3/1
  Bus Selector3/1 -> [MTR_TWtrOut_degC]  "<MTR_TWtrOutRr_degC>"
  [MTR_TWtrOut_degC] -> Low Temperature Radiator/1(MTR_TWtrOut_degC)
  [RAD_TWtrOut_degC] -> Bus Creator/2  "PTCS_TWtrOut_degC"
  [RAD_PHeatRej_W] -> Bus Creator/3  "PTCS_PHeatRejRad_W"
  Bus Selector1/1 -> [INIT_TSys_degC]  "<INIT_TSys_degC>"
  Delay/1 -> [RAD_TWtrOut_degC]
  [INIT_TSys_degC] -> Delay/2
  [MTR_TWtrOut_degC] -> Bus Creator/1  "PTCS_TWtrIn_degC"
  [VCU_rFlowMtrRr] -> Divide6/2
  Divide6/1 -> [RAD_dVPwrTRr_lpm]
  [VCU_rFlowMtrFr] -> Divide5/2
  Divide5/1 -> [RAD_dVPwrTFrt_lpm]
  Bus Selector4/1 -> [VCU_rFlowMtrFr]  "<VCU_rFlowMtrFr>"
  VCU/1 -> Bus Selector4/1
  Bus Selector4/2 -> [VCU_rFlowMtrRr]  "<VCU_rFlowMtrRr>"
  Bus Selector4/3 -> [VCU_dVPwrT_lpm]  "<VCU_dVPwrT_lpm>"
  [RAD_dVPwrTFrt_lpm] -> Add/1
  [RAD_dVPwrTRr_lpm] -> Add/2
  Add/1 -> [RAD_dVPwr_lpm]
  [RAD_dVPwrTRr_lpm] -> Bus Creator/6  "PTCS_dVPwrTRr_lpm"
  [RAD_dVPwrTFrt_lpm] -> Bus Creator/5  "PTCS_dVPwrTFrt_lpm"
  [RAD_dVPwr_lpm] -> Bus Creator/4  "PTCS_dVPwrT_lpm"
  Low Temperature Radiator/1(RAD_TWtrOut_degC) -> Delay/1
  Low Temperature Radiator/2(RAD_PHeatRej_W) -> [RAD_PHeatRej_W]
  BCS/1 -> Bus Selector5/1
  Bus Selector5/1 -> [RADBCS_TAirOut_degC]  "<BCS_TAirOut_degC>"
  Bus Selector2/1 -> [RAD_dmAir_kgps]  "<RAD_dmAir_kgps>"
  Bus Selector2/2 -> [RAD_VAirTot_mps]  "<RAD_VAirTot_mps>"
  FAN/1 -> Bus Selector2/1
  [RAD_VAirTot_mps] -> Low Temperature Radiator/5(RAD_vAir_mps)
  [VCU_dVPwrT_lpm] -> Pump Input Power [W]/1, Pump Inertia/1(VCU_dVBtr_lpm)
  Pump Input Power [W]/1 -> [PTCS_PumpPwr_W]
  [PTCS_PumpPwr_W] -> Bus Creator/7  "PTCS_PumpPwr_W"
  Pump Inertia/1(BCS_dV_lpm) -> Divide6/1, Divide5/1

== system Vehicle_Model_WIP_V2/VCU/Torque Distribution/TractionControl ==
  slipFr : Inport
  sensors : Inport  Port=2
  slipRr : Inport  Port=3
  Add : Sum  Inputs=|+-
  Add1 : Sum  Inputs=|+-
  Bus Selector : BusSelector  OutputSignals=traction,TrqReqFr,TrqReqRr
  Gain : Gain  Gain=0.1
  Mux : Mux  Inputs=2
  Mux1 : Mux  Inputs=2
  PID Controller : simulink/Continuous/PID Controller  Controller=PID  Form=Parallel  TimeDomain=Discrete-time  SampleTime=-1  IntegratorMethod=Forward Euler  FilterMethod=Forward Euler  ControllerParametersSource=internal  P=VHCL.TC_P*0.5  I=0  D=0.1  UseFilter=on  N=80  TunerSelectOption=Transfer Function Based (PID Tuner App)  InitialConditionSource=internal  InitialConditionForIntegrator=0  InitialConditionForFilter=0  DifferentiatorICPrevScaledInput=0  ExternalReset=none  TrackingMode=off  Kt=1  LimitOutput=off  UpperSaturationLimit=inf  LowerSaturationLimit=-inf  LinearizeAsGain=on  AntiWindupMode=none  Kb=1  POutMin=[]  POutMax=[]  IOutMin=[]  IOutMax=[]  DOutMin=[]  DOutMax=[]  NOutMin=[]  NOutMax=[]  SumOutMin=[]  SumOutMax=[]  SaturationOutMin=[]  SaturationOutMax=[]  PParamMin=[]  PParamMax=[]  IParamMin=[]  IParamMax=[]  DParamMin=[]  DParamMax=[]  NParamMin=[]  NParamMax=[]  KbParamMin=[]  KbParamMax=[]  KtParamMin=[]  KtParamMax=[]  KbOutMin=[]  KbOutMax=[]  KtOutMin=[]  KtOutMax=[]  IntegratorOutMin=[]  IntegratorOutMax=[]  FilterOutMin=[]  FilterOutMax=[]  SumI1OutMin=[]  SumI1OutMax=[]  SumI2OutMin=[]  SumI2OutMax=[]  SumI3OutMin=[]  SumI3OutMax=[]  SumI4OutMin=[]  SumI4OutMax=[]  SumDOutMin=[]  SumDOutMax=[]  DifferentiatorOutMin=[]  DifferentiatorOutMax=[]  FilterDiffOutCoefMin=[]  FilterDiffOutCoefMax=[]  ReciprocalOutMin=[]  ReciprocalOutMax=[]  SumDenOutMin=[]  SumDenOutMax=[]  SumNumOutMin=[]  SumNumOutMax=[]  DivideOutMin=[]  DivideOutMax=[]  IntegratorContinuousStateAttributes=''  IntegratorStateMustResolveToSignalObject=off  IntegratorRTWStateStorageClass=Auto  FilterContinuousStateAttributes=''  FilterStateMustResolveToSignalObject=off  FilterRTWStateStorageClass=Auto  ParallelPVariant=InternalParameters  IdealPVariant=Disabled  IVariant=InternalParameters  DVariant=InternalParameters  IntegratorVariant=Discrete  SatVariant=Disabled  AWVariant=Passthrough  PCopyVariant=Disabled  TRVariant=Disabled  FdbkBlocksVariant=Forward  IdealPFdbkVariant=Disabled  SatFdbkVariant=Disabled  DerivativeFilterVariant=ForwardEulerFilter  NVariant=InternalParameters  NCopyVariant=Disabled  FilterICVariant=InternalICsFilter  IntegratorICVariant=InternalICs  ExternalResetVariant=Disabled  TRSumVariant=Passthrough  SumFdbkVariant=Disabled  SumVariant=Sum_PID
  PID Controller1 : simulink/Continuous/PID Controller  Controller=PID  Form=Parallel  TimeDomain=Discrete-time  SampleTime=-1  IntegratorMethod=Forward Euler  FilterMethod=Forward Euler  ControllerParametersSource=internal  P=VHCL.TC_P  I=0  D=0.1  UseFilter=on  N=80  TunerSelectOption=Transfer Function Based (PID Tuner App)  InitialConditionSource=internal  InitialConditionForIntegrator=0  InitialConditionForFilter=0  DifferentiatorICPrevScaledInput=0  ExternalReset=none  TrackingMode=off  Kt=1  LimitOutput=off  UpperSaturationLimit=inf  LowerSaturationLimit=-inf  LinearizeAsGain=on  AntiWindupMode=none  Kb=1  POutMin=[]  POutMax=[]  IOutMin=[]  IOutMax=[]  DOutMin=[]  DOutMax=[]  NOutMin=[]  NOutMax=[]  SumOutMin=[]  SumOutMax=[]  SaturationOutMin=[]  SaturationOutMax=[]  PParamMin=[]  PParamMax=[]  IParamMin=[]  IParamMax=[]  DParamMin=[]  DParamMax=[]  NParamMin=[]  NParamMax=[]  KbParamMin=[]  KbParamMax=[]  KtParamMin=[]  KtParamMax=[]  KbOutMin=[]  KbOutMax=[]  KtOutMin=[]  KtOutMax=[]  IntegratorOutMin=[]  IntegratorOutMax=[]  FilterOutMin=[]  FilterOutMax=[]  SumI1OutMin=[]  SumI1OutMax=[]  SumI2OutMin=[]  SumI2OutMax=[]  SumI3OutMin=[]  SumI3OutMax=[]  SumI4OutMin=[]  SumI4OutMax=[]  SumDOutMin=[]  SumDOutMax=[]  DifferentiatorOutMin=[]  DifferentiatorOutMax=[]  FilterDiffOutCoefMin=[]  FilterDiffOutCoefMax=[]  ReciprocalOutMin=[]  ReciprocalOutMax=[]  SumDenOutMin=[]  SumDenOutMax=[]  SumNumOutMin=[]  SumNumOutMax=[]  DivideOutMin=[]  DivideOutMax=[]  IntegratorContinuousStateAttributes=''  IntegratorStateMustResolveToSignalObject=off  IntegratorRTWStateStorageClass=Auto  FilterContinuousStateAttributes=''  FilterStateMustResolveToSignalObject=off  FilterRTWStateStorageClass=Auto  ParallelPVariant=InternalParameters  IdealPVariant=Disabled  IVariant=InternalParameters  DVariant=InternalParameters  IntegratorVariant=Discrete  SatVariant=Disabled  AWVariant=Passthrough  PCopyVariant=Disabled  TRVariant=Disabled  FdbkBlocksVariant=Forward  IdealPFdbkVariant=Disabled  SatFdbkVariant=Disabled  DerivativeFilterVariant=ForwardEulerFilter  NVariant=InternalParameters  NCopyVariant=Disabled  FilterICVariant=InternalICsFilter  IntegratorICVariant=InternalICs  ExternalResetVariant=Disabled  TRSumVariant=Passthrough  SumFdbkVariant=Disabled  SumVariant=Sum_PID
  Product{,1..5} (6 alike) : Product
  Saturation : Saturate  UpperLimit=1  LowerLimit=0
  Saturation1 : Saturate  UpperLimit=1  LowerLimit=0
  Scope : Scope  NumInputPorts=2
  Sign : Signum
  Sign1 : Signum
  Subtract : Sum
  Subtract1 : Sum
  targetSlipFr : Constant  Value=0.125
  targetSlipRr : Constant  Value=0.125
  TCTrqReqFr : Outport
  TCTrqReqRr : Outport  Port=2
  wires:
  sensors/1 -> Bus Selector/1
  Bus Selector/1 -> [traction]  "<traction>"
  Product1/1 -> Add/1
  slipFr/1 -> Add/2
  Add/1 -> PID Controller/1
  Sign1/1 -> Subtract/1, Product1/1
  slipRr/1 -> Add1/2
  Product/1 -> Add1/1
  targetSlipRr/1 -> Product/2
  Sign/1 -> Subtract1/1, Product/1
  [TrqReqFr] -> Sign1/1
  targetSlipFr/1 -> Product1/2
  Product2/1 -> Subtract/2
  Add1/1 -> PID Controller1/1
  Product3/1 -> Subtract1/2
  [TrqReqRr] -> Sign/1
  [TrqReqRr] -> Mux/1, Product4/2  "TrqReqRr"
  [TrqReqFr] -> Mux1/1, Product5/1  "TrqReqFr"
  Subtract/1 -> Saturation/1
  Subtract1/1 -> Saturation1/1
  Mux/1 -> Scope/2
  Mux1/1 -> Scope/1
  [traction] -> Gain/1
  Saturation/1 -> Product5/2
  Saturation1/1 -> Product4/1
  PID Controller/1 -> Product2/1
  PID Controller1/1 -> Product3/2
  Gain/1 -> Product2/2, Product3/1
  Bus Selector/3 -> [TrqReqRr]  "<TrqReqRr>"
  Bus Selector/2 -> [TrqReqFr]  "<TrqReqFr>"
  Product5/1 -> Mux1/2, TCTrqReqFr/1  "TCTrqReqFr"
  Product4/1 -> Mux/2, TCTrqReqRr/1  "TCTrqReqRr"

== system Vehicle_Model_WIP_V2/VCU/Torque Distribution/TrqDistr ==
  TCTrqReqFr : Inport
  RWheelFr : Inport  Port=2
  WDistrFr : Inport  Port=3
  sensors : Inport  Port=4
  WDistrRr : Inport  Port=5
  RWheelRr : Inport  Port=6
  TCTrqReqRr : Inport  Port=7
  Bus Selector : BusSelector  OutputSignals=TrqReqFr,TrqReqRr
  Bus Selector1 : BusSelector  OutputSignals=traction
  Constant1 : Constant  Value=MTR.Front.Number_of_Motors
  Constant2 : Constant  Value=MTR.Rear.Number_of_Motors
  Constant4 : Constant  Value=TRSM.Front.Trans_Tau
  Constant5 : Constant  Value=TRSM.Rear.Trans_Tau
  Discrete Filter : DiscreteFilter  Numerator=[0.2]  Denominator=[1 -0.8]
  Discrete Filter1 : DiscreteFilter  Numerator=[0.2]  Denominator=[1 -0.8]
  Gain : Gain  Gain=1.1
  Gain1 : Gain  Gain=1.1
  Gain2 : Gain  Gain=-1.1
  Gain3 : Gain  Gain=-1.1
  If : If  IfExpression=u1 == 0
  If Action Subsystem : Subsystem  TreatAsAtomicUnit=on
  If Action Subsystem1 : Subsystem  TreatAsAtomicUnit=on
  Merge : Merge
  Merge1 : Merge
  Mux{,1..3} (4 alike) : Mux  Inputs=2
  Product1 : Product  Inputs=/***
  Product11 : Product  Inputs=/*
  Product12 : Product  Inputs=*/
  Product2 : Product  Inputs=***/
  Saturation Dynamic : simulink/Discontinuities/Saturation Dynamic  OutMin=[]  OutMax=[]  OutDataTypeStr=Inherit: Same as second input  OutDataType=fixdt(1, 16)  OutScaling=2^-10  DoSatur=off
  Saturation Dynamic1 : simulink/Discontinuities/Saturation Dynamic  OutMin=[]  OutMax=[]  OutDataTypeStr=Inherit: Same as second input  OutDataType=fixdt(1, 16)  OutScaling=2^-10  DoSatur=off
  Scope : Scope  NumInputPorts=2
  mi1 : Constant  Value=VHCL.Front.mu
  mi2 : Constant  Value=VHCL.Rear.mu
  INVTrqReqFr : Outport
  DstrTrqReqFr : Outport  Port=2
  INVTrqReqRr : Outport  Port=3
  DstrTrqReqRr : Outport  Port=4
  wires:
  Constant2/1 -> Product1/1
  Constant1/1 -> Product2/4
  RWheelRr/1 -> Product1/3
  WDistrRr/1 -> Discrete Filter1/1
  WDistrFr/1 -> Discrete Filter/1
  RWheelFr/1 -> Product2/2
  Bus Selector/1 -> [TFr0]  "<TrqReqFr>"
  Product2/1 -> Product11/2
  Product1/1 -> Product12/1
  sensors/1 -> [sensors]
  [sensors] -> Bus Selector/1
  [sensors] -> Bus Selector1/1
  Bus Selector1/1 -> If/1  "<traction>"
  If/2 -> If Action Subsystem/Action
  TCTrqReqRr/1 -> If Action Subsystem/2(TCRr)
  TCTrqReqFr/1 -> If Action Subsystem/1(TCFr)
  If/1 -> If Action Subsystem1/Action
  If Action Subsystem1/1(Out1) -> Merge/1
  If Action Subsystem1/2(Out2) -> Merge1/1
  Merge/1 -> INVTrqReqFr/1
  Merge1/1 -> INVTrqReqRr/1
  Bus Selector/2 -> [TRr0]  "<TrqReqRr>"
  Saturation Dynamic/1 -> Mux3/2, DstrTrqReqRr/1, If Action Subsystem1/2(In2)  "DistrTrqReqRr"
  Saturation Dynamic1/1 -> If Action Subsystem1/1(In1), Mux2/2, DstrTrqReqFr/1  "DistrTrqReqFr"
  Discrete Filter/1 -> Product2/3
  Discrete Filter1/1 -> Product1/2
  If Action Subsystem/1(Fr) -> Merge/2
  If Action Subsystem/2(Rr) -> Merge1/2
  mi1/1 -> Product2/1
  mi2/1 -> Product1/4
  Constant4/1 -> Product11/1
  Constant5/1 -> Product12/2
  Product11/1 -> [MxTrqFrt]
  Product12/1 -> [MxTrqRr]
  [TFr0] -> Mux/2, Saturation Dynamic1/2
  [TRr0] -> Mux1/2, Saturation Dynamic/2
  [MxTrqFrt] -> Gain/1
  [MxTrqFrt] -> Gain2/1
  [MxTrqRr] -> Gain1/1
  [MxTrqRr] -> Gain3/1
  Gain/1 -> Mux/1, Saturation Dynamic1/1
  Gain1/1 -> Saturation Dynamic/1, Mux1/1
  Gain2/1 -> Saturation Dynamic1/3
  Gain3/1 -> Saturation Dynamic/3
  Mux/1 -> Mux2/1
  Mux1/1 -> Mux3/1
  Mux3/1 -> Scope/2
  Mux2/1 -> Scope/1

== system Vehicle_Model_WIP_V2/VCU/Torque Distribution/sensors PREPROCESS ==
  sensors_IO : Inport
  TrqReqFr : Inport  Port=2
  TrqReqRr : Inport  Port=3
  Bus Creator : BusCreator  Inputs=3
  Saturation : Saturate  UpperLimit=20  LowerLimit=0
  sensors : Outport
  wires:
  TrqReqRr/1 -> Bus Creator/3  "TrqReqRr"
  TrqReqFr/1 -> Bus Creator/2  "TrqReqFr"
  sensors_IO/1 -> Saturation/1
  Bus Creator/1 -> sensors/1
  Saturation/1 -> Bus Creator/1  "traction"

== system Vehicle_Model_WIP_V2/VCU/Torque Request/Regen ==
  DRV_rBrake : Inport
  VLD_vAct : Inport  Port=2
  TrqDistrFr : Inport  Port=3
  1-D Lookup Table : Lookup_n-D  NumberOfTableDimensions=1  BreakpointsForDimension1=[0 5 10 100]  Table=[0 0 1 1]  InternalRulePriority=Speed  RndMeth=Simplest  InputSameDT=on
  Constant : Constant  Value=BRK.Front.Mx_Torque_Nm
  Constant1 : Constant  Value=TRSM.Front.Trans_Tau
  Constant2 : Constant  Value=BRK.Rear.Mx_Torque_Nm
  Constant4 : Constant  Value=TRSM.Rear.Trans_Tau
  Gain : Gain  Gain=0.5
  Gain1 : Gain  Gain=MTR.Front.Number_of_Motors
  Gain2 : Gain  Gain=MTR.Rear.Number_of_Motors
  Product1 : Product  Inputs=*/
  Product2 : Product  Inputs=/*
  Product3 : Product  Inputs=**
  Product4 : Product  Inputs=**
  Product5 : Product
  Saturation1 : Saturate  UpperLimit=0  LowerLimit=-Simulink.INIT_rRegen*0.28*(VHCL.tot_mass_kg+VHCL.Towing_w_kg)*9.81*0.36/(BRK.Front.Mx_Torque_Nm+BRK.Rear.Mx_Torque_Nm)
  Scope : Scope  NumInputPorts=2
  Subtract1 : Sum  Inputs=-+
  Sum1 : Sum
  Sum3 : Sum  Inputs=+-
  BrkTrqReqFr : Outport
  BrkTrqReqRr : Outport  Port=2
  rBrk : Outport  Port=3
  wires:
  VLD_vAct/1 -> 1-D Lookup Table/1
  TrqDistrFr/1 -> Product3/2
  DRV_rBrake/1 -> Subtract1/2, Saturation1/1
  Subtract1/1 -> rBrk/1
  Saturation1/1 -> Product5/2
  Product5/1 -> Gain/1, Subtract1/1
  1-D Lookup Table/1 -> Product5/1
  [rMtr] -> Sum3/1, Product3/1
  Product3/1 -> Product1/1, Sum3/2
  Product1/1 -> Scope/2, BrkTrqReqFr/1
  Sum3/1 -> Product2/2
  Product2/1 -> BrkTrqReqRr/1, Scope/1
  Constant1/1 -> Product1/2
  Constant4/1 -> Product2/1
  Gain/1 -> Product4/2
  Sum1/1 -> Product4/1
  Product4/1 -> [rMtr]
  Gain2/1 -> Sum1/2  "Torque request [Nm]"
  Gain1/1 -> Sum1/1  "Torque request [Nm]"
  Constant2/1 -> Gain2/1
  Constant/1 -> Gain1/1

== system Vehicle_Model_WIP_V2/VCU/Torque Request/TrqDstr ==
  DRV_rThrottle : Inport
  TrqDistrFr : Inport  Port=2
  Constant : Constant  Value=MTR.Front.Max_Torque_Nm
  Constant1 : Constant  Value=MTR.Rear.Max_Torque_Nm
  Gain : Gain
  Gain1 : Gain  Gain=MTR.Front.Number_of_Motors
  Gain2 : Gain  Gain=MTR.Rear.Number_of_Motors
  Product1 : Product
  Product3 : Product
  Scope : Scope  NumInputPorts=2
  Sum : Sum
  Sum1 : Sum  Inputs=+-
  TrqReqFr : Outport
  TrqReqRr : Outport  Port=2
  wires:
  DRV_rThrottle/1 -> [DRV_rThrottle]
  Constant1/1 -> Gain2/1
  Constant/1 -> Gain1/1
  Sum/1 -> Gain/1
  [DRV_rThrottle] -> Product3/2
  Product3/1 -> Sum1/1, Product1/1
  [TrqDstrbFr] -> Product1/2
  Product1/1 -> Sum1/2, Scope/2, TrqReqFr/1
  Sum1/1 -> Scope/1, TrqReqRr/1
  Gain/1 -> Product3/1
  TrqDistrFr/1 -> [TrqDstrbFr]
  Gain1/1 -> Sum/1  "Torque request [Nm]"
  Gain2/1 -> Sum/2  "Torque request [Nm]"

== system Vehicle_Model_WIP_V2/VLD/Front Wheel Radius/ Wheel static radius under load ==
  Add1 : Sum
  Constant : Constant  Value=VHCL.Front.Rim_diam_inch
  Constant1 : Constant  Value=1000
  Constant2 : Constant  Value=VHCL.Front.Shoulder_perc
  Constant3 : Constant  Value=VHCL.Front.Tyre_Width_mm
  Constant4 : Constant  Value=100
  Constant5 : Constant  Value=2
  Constant6 : Constant  Value=0.0254
  Constant7 : Constant  Value=0.95
  Divide1 : Product  Inputs=*/
  Divide10 : Product
  Divide2 : Product  Inputs=*/
  Divide3 : Product  Inputs=*/
  Divide8 : Product
  Divide9 : Product
  LVD_RFrStc_m : Outport  VectorParamsAs1DForOutWhenUnconnected=off
  wires:
  Constant3/1 -> Divide3/1
  Constant1/1 -> Divide3/2
  Constant2/1 -> Divide1/1
  Constant4/1 -> Divide1/2
  Constant/1 -> Divide2/1
  Constant5/1 -> Divide2/2
  Divide2/1 -> Divide8/1
  Constant6/1 -> Divide8/2
  Divide3/1 -> Divide9/1
  Divide1/1 -> Divide9/2
  Divide9/1 -> Add1/1
  Divide8/1 -> Add1/2
  Add1/1 -> Divide10/1
  Constant7/1 -> Divide10/2
  Divide10/1 -> LVD_RFrStc_m/1

== system Vehicle_Model_WIP_V2/VLD/Rear Wheel Radius/ Wheel static radius under load ==
  Add1 : Sum
  Constant : Constant  Value=VHCL.Front.Rim_diam_inch
  Constant1 : Constant  Value=1000
  Constant2 : Constant  Value=VHCL.Front.Shoulder_perc
  Constant3 : Constant  Value=VHCL.Front.Tyre_Width_mm
  Constant4 : Constant  Value=100
  Constant5 : Constant  Value=2
  Constant6 : Constant  Value=0.0254
  Constant7 : Constant  Value=0.95
  Divide1 : Product  Inputs=*/
  Divide10 : Product
  Divide2 : Product  Inputs=*/
  Divide3 : Product  Inputs=*/
  Divide8 : Product
  Divide9 : Product
  LVD_RFrStc_m : Outport  VectorParamsAs1DForOutWhenUnconnected=off
  wires:
  Constant3/1 -> Divide3/1
  Constant1/1 -> Divide3/2
  Constant2/1 -> Divide1/1
  Constant4/1 -> Divide1/2
  Constant/1 -> Divide2/1
  Constant5/1 -> Divide2/2
  Divide2/1 -> Divide8/1
  Constant6/1 -> Divide8/2
  Divide3/1 -> Divide9/1
  Divide1/1 -> Divide9/2
  Divide9/1 -> Add1/1
  Divide8/1 -> Add1/2
  Add1/1 -> Divide10/1
  Constant7/1 -> Divide10/2
  Divide10/1 -> LVD_RFrStc_m/1
